simulink model "Controller4"  (Simulink 6.5)
settings: Solver=ode3  StartTime=0.0  StopTime=400  FixedStep=0.1  RelTol=1e-3
settings Model: Creator=Andres Toom  LastModifiedBy=naks
settings OptimizationCC: InitFltsAndDblsToZero=off  OptimizeModelRefInitCode=on  LifeSpan=1
settings DebuggingCC: SignalResolutionControl=UseLocalSettings
settings RTWCC: SystemTargetFile=ert.tlc  TemplateMakefile=ert_default_tmf  Description=Real-Time Workshop Embedded Coder (no auto configuration)  ProcessScript=ert_make_rtw_hook
settings CodeAppCC: IgnoreCustomStorageClasses=off
settings ERTTargetCC: TargetFcnLib=ansi_tfl_tmw.mat  GenFloatMathFcnCalls=ANSI_C  GenerateSampleERTMain=on  InlinedParameterPlacement=NonHierarchical  ERTCustomFileTemplate=example_file_process.tlc

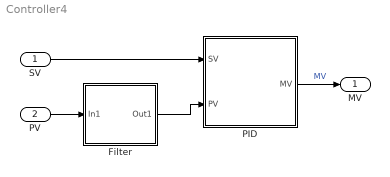
== system Controller4 ==
  SV : Inport  PortDimensions=1  DataType=double  OutDataType=fixdt(1,16,0)  OutScaling=[]
  PV : Inport  Port=2  PortDimensions=1  DataType=double  OutDataType=fixdt(1,16,0)  OutScaling=[]
  Filter : Subsystem
  PID : Subsystem  TreatAsAtomicUnit=on
  MV : Outport  OutDataType=fixdt(1,16,0)  OutScaling=[]
  wires:
  Filter/1(Out1) -> PID/2(PV)
  SV/1 -> PID/1(SV)
  PV/1 -> Filter/1(In1)
  PID/1(MV) -> MV/1  "MV"

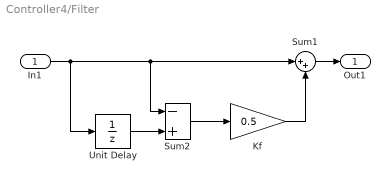
== system Controller4/Filter ==
  In1 : Inport  OutDataType=fixdt(1,16,0)  OutScaling=[]
  Kf : Gain  Gain=0.5
  Sum1 : Sum  Inputs=|++
  Sum2 : Sum  Inputs=|-+
  Unit Delay : UnitDelay  SampleTime=-1
  Out1 : Outport  OutDataType=fixdt(1,16,0)  OutScaling=[]
  wires:
  In1/1 -> Unit Delay/1, Sum1/1, Sum2/1
  Kf/1 -> Sum1/2
  Unit Delay/1 -> Sum2/2
  Sum2/1 -> Kf/1
  Sum1/1 -> Out1/1

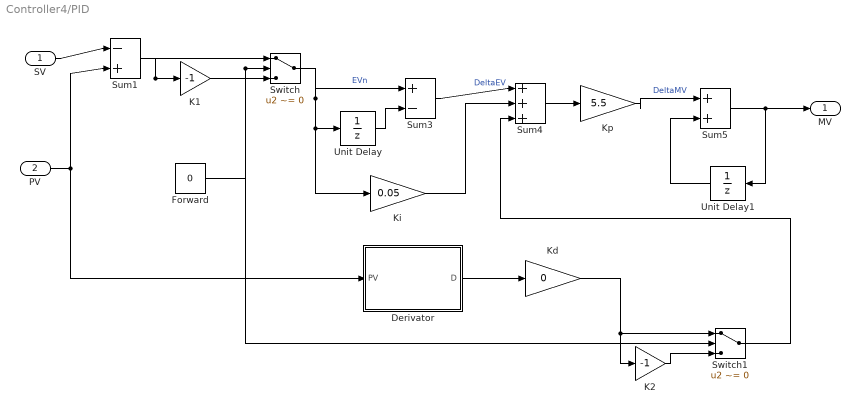
== system Controller4/PID ==
  SV : Inport  OutDataType=fixdt(1,16,0)  OutScaling=[]
  PV : Inport  Port=2  OutDataType=fixdt(1,16,0)  OutScaling=[]
  Derivator : Subsystem  TreatAsAtomicUnit=on
  Forward : Constant  Value=0  OutDataType=sfix(16)  ConRadixGroup=Use specified scaling  OutScaling=2^0  SampleTime=inf  FramePeriod=inf
  K1 : Gain  Gain=-1
  K2 : Gain  Gain=-1
  Kd : Gain  Gain=0
  Ki : Gain  Gain=0.05
  Kp : Gain  Gain=5.5
  Sum1 : Sum  Inputs=|-+
  Sum3 : Sum  Inputs=|+-
  Sum4 : Sum  Inputs=|+++
  Sum5 : Sum  Inputs=|++
  Switch : Switch  Criteria=u2 ~= 0
  Switch1 : Switch  Criteria=u2 ~= 0
  Unit Delay : UnitDelay  SampleTime=-1
  Unit Delay1 : UnitDelay  Orientation=left  SampleTime=-1
  MV : Outport  OutDataType=fixdt(1,16,0)  OutScaling=[]
  wires:
  SV/1 -> Sum1/1
  PV/1 -> Sum1/2, Derivator/1(PV)
  Sum1/1 -> Switch/1, K1/1
  Forward/1 -> Switch/2, Switch1/2
  Switch/1 -> Sum3/1, Unit Delay/1, Ki/1  "EVn"
  Unit Delay/1 -> Sum3/2
  Sum3/1 -> Sum4/1  "DeltaEV"
  Sum4/1 -> Kp/1
  Sum5/1 -> MV/1, Unit Delay1/1
  Kp/1 -> Sum5/1  "DeltaMV"
  Unit Delay1/1 -> Sum5/2
  Ki/1 -> Sum4/2
  Switch1/1 -> Sum4/3
  K1/1 -> Switch/3
  K2/1 -> Switch1/3
  Derivator/1(D) -> Kd/1
  Kd/1 -> K2/1, Switch1/1

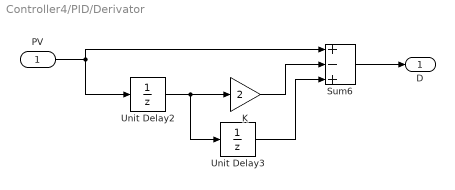
== system Controller4/PID/Derivator ==
  PV : Inport  OutDataType=fixdt(1,16,0)  OutScaling=[]
  K : Gain  Gain=2
  Sum6 : Sum  Inputs=|+-+
  Unit Delay2 : UnitDelay  SampleTime=-1
  Unit Delay3 : UnitDelay  SampleTime=-1
  D : Outport  OutDataType=fixdt(1,16,0)  OutScaling=[]
  wires:
  Sum6/1 -> D/1
  Unit Delay2/1 -> Unit Delay3/1, K/1
  Unit Delay3/1 -> Sum6/3
  K/1 -> Sum6/2
  PV/1 -> Unit Delay2/1, Sum6/1
